simulink model "KinematischesModell_Rover"  (R2024a)
settings: Solver=VariableStepAuto  StartTime=0.0  StopTime=simTime  RelTol=1e-3
values from neighbouring files (symbols this model uses):
  roverWidth = 0.4    [Initialisierung_Rover_.m]
  wheelRadius = 0.1    [Initialisierung_Rover_.m]
undefined symbols (not defined in the file or in its folder): qstart
settings Model: Creator=Asus  LastModifiedBy=Asus

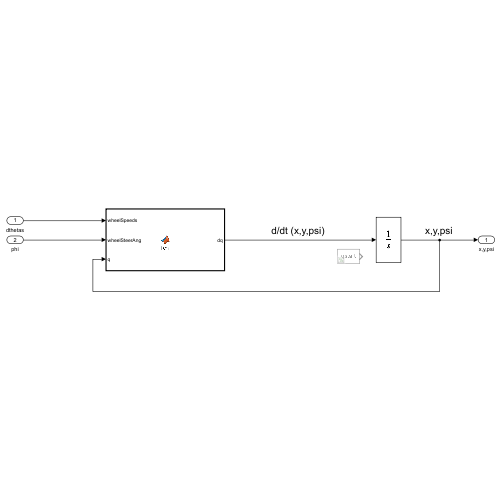
[thumbnail: Simulink's stored preview of the top-level diagram]
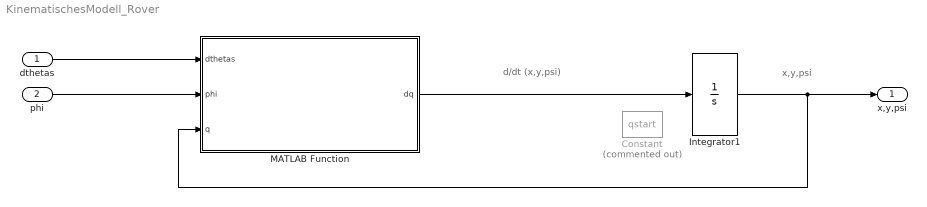
== system KinematischesModell_Rover ==
  note: d/dt (x,y,psi)
  note: x,y,psi
  dthetas : Inport
  phi : Inport  Port=2
  Constant : Constant  Commented=on  Value=qstart
  Integrator1 : Integrator
  MATLAB Function : MATLAB Function  TreatAsAtomicUnit=on
  x,y,psi : Outport
  wires:
  dthetas/1 -> MATLAB Function/1(dthetas)
  phi/1 -> MATLAB Function/2(phi)
  MATLAB Function/1(dq) -> Integrator1/1
  Integrator1/1 -> MATLAB Function/3(q), x,y,psi/1

== matlab function KinematischesModell_Rover/MATLAB Function ==
  data: dthetas input; phi input; q input; dq output; wheelRadius parameter; roverWidth parameter
function dq = fcn(dthetas, phi, q, wheelRadius, roverWidth)

% wenn wheelRadius kein input ist, kommt es dann aus der Workspace?

psi = q(3); 

dq = zeros(3,1);

% Rotationsmatrix
Rz = [cos(psi) -sin(psi) 0;
    sin(psi) cos(psi) 0;
    0 0 1];

% Lokale Geschwindigkeiten
vx = (wheelRadius/4) * (dthetas(1)*cos(phi(1)) + dthetas(2)*cos(phi(2)) + ...
                        dthetas(3)*cos(phi(3)) + dthetas(4)*cos(phi(4))); 

vy = (wheelRadius/4) * (dthetas(1)*sin(phi(1)) + dthetas(2)*sin(phi(2)) + ...
                        dthetas(3)*sin(phi(3)) + dthetas(4)*sin(phi(4)));

omega = (wheelRadius/2*roverWidth) * (dthetas(1)*cos(phi(1)) - dthetas(2)*cos(phi(2)) - ...
                        dthetas(3)*cos(phi(3)) + dthetas(4)*cos(phi(4)));

roverSpeedLoc = [vx vy omega]';

dq = Rz*roverSpeedLoc;
